simulink model "receiver_overall_reset"  (Simulink 7.5)
settings: Solver=FixedStepDiscrete  SolverMode=SingleTasking  StartTime=0.0  StopTime=(length(simin.signals.values)-1)/Fs  FixedStep=1  RelTol=1e-3
undefined symbols (not defined in the file): Fs
libraries: xbsIndex_r4 x962
(part 1 of 9)
settings Model: Creator=ich  LastModifiedBy=ich
settings DataIOCC: ExternalInput=simin  LimitDataPoints=off  LoadExternalInput=on

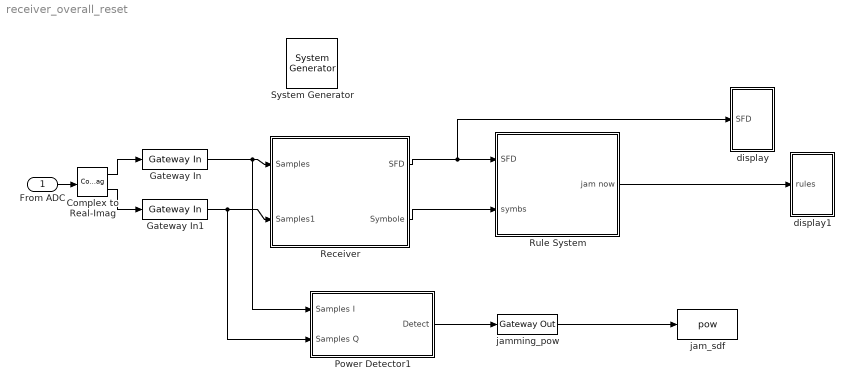
== system receiver_overall_reset ==
  From ADC : Inport  SampleTime=1/Fs  OutDataType=fixdt(1, 16)  OutScaling=2^0  Interpolate=off
      settings: SignalType=complex
  " System Generator" : xbsIndex_r4/ System Generator  Tag=genX  SystemSampleTime=-1  xilinxfamily=spartan3  part=xc3s2000  speed=-5  package=fg456  synthesis_tool=XST  clock_wrapper=Clock Enables  directory=G:/Projekte/wireless_firewall/dschung/IEEE 802.15.4 receiver/receiver_overall_reset  testbench=off  simulink_period=1  sysclk_period=10  dcm_input_clock_period=10  incr_netlist=off  trim_vbits=Everywhere in SubSystem  dbl_ovrd=According to Block Masks  core_generation=According to Block Masks  run_coregen=off  deprecated_control=off  eval_field=0  block_type=sysgen
      settings: block_version=12.1
  Complex to Real-Imag : ComplexToRealImag
  Gateway In : xbsIndex_r4/Gateway In  arith_type="Signed  (2's comp)"  n_bits=15  bin_pt=13  quantization="Round  (unbiased: +/- Inf)"  overflow=Saturate  period=1/Fs  dbl_ovrd=off  timing_constraint=None  locs_specified=off  LOCs={}  hdl_port=on  block_type=gatewayin
      settings: infoedit="Gateway in block.  Converts inputs of type Simulink integer, double and fixed point to  Xilinx fixed point type.<br><br>Hardware notes:  In hardware these blocks become top level input ports."  xl_area=[0 0 0 0 16 0 0]  block_version=12.1
  Gateway In1 : xbsIndex_r4/Gateway In  arith_type="Signed  (2's comp)"  n_bits=15  bin_pt=13  quantization="Round  (unbiased: +/- Inf)"  overflow=Saturate  period=1/Fs  dbl_ovrd=off  timing_constraint=None  locs_specified=off  LOCs={}  hdl_port=on  block_type=gatewayin
      settings: infoedit="Gateway in block.  Converts inputs of type Simulink integer, double and fixed point to  Xilinx fixed point type.<br><br>Hardware notes:  In hardware these blocks become top level input ports."  xl_area=[0 0 0 0 16 0 0]  block_version=12.1
  Power Detector1 : Subsystem
  Receiver : Subsystem
  Rule System : Subsystem  mask{head=4, s16a=0, spl=0, spu=0, s16l=0, s16u=0, d16a=0, dpl=0, dpu=0, d16l=0, d16u=0, b64a=0, d64lr=0, d64ll=0, d64ur=0, d64ul=0, s64lr=0, s64ll=0, s64ur=0, s64ul=0}
      mask prompts: head "Header Jam Type"; s16a "Source 16 bit Address"; spl "Source PAN lower"; spu "Source PAN upper"; s16l "Source 16 bit lower"; s16u "Source 16 bit upper"; d16a "Dest 16bit Address"; dpl "Dest PAN lower"; dpu "Dest PAN upper"; d16l "Dest 16 bit lower"; d16u "Dest 16 bit upper"; b64a "64 bit add jamming"; d64lr "Dest 64 bit lower rigth part"; d64ll "Dest 64 bit lower left part"; d64ur "Dest 64 bit upper rigth part"; d64ul "Dest 64 bit upper left part"; s64lr "Source 64 bit lower rigth part"; s64ll "Source 64 bit lower left part"; s64ur "Source 64 bit upper rigth part"; s64ul "Source 64 bit upper left part"
      mask help:
      | head:
      |   first bit: security
      |   second bit: is Beacon
      |   third bit: is MAC
      | Dest + Source 16 Addresses:
      |   first bit: PAN
      |   second bit: Address
      |  Addresses with MSB rigth!
      | 64 bit Addresses:
      |   first bit: Destination
      |   second bit: Source
      |  Addresses with MSB rigth!
      |  Bsp: 123456789ABCDEFG0 -->
      |    rigth: '87654321'
      |    left:  '0FEDCBA9'
  display : Subsystem
  display1 : Subsystem
  jam_sdf : ToWorkspace  VariableName=pow  SampleTime=-1  SaveFormat=Structure
  jamming_pow : xbsIndex_r4/Gateway Out  hdl_port=on  timing_constraint=None  locs_specified=off  LOCs={}  block_type=gatewayout
      settings: infoedit="Gateway out block.  Converts Xilinx fixed point inputs into ouputs of type Simulink integer, double, or fixed point.<br><br>Hardware notes:  In hardware these blocks become top level output ports or are discarded, depending on how they are configured."  block_version=12.2
  wires:
  Receiver/2(Symbole) -> Rule System/2(symbs)
  Receiver/1(SFD) -> Rule System/1(SFD), display/1(SFD)
  Rule System/1(jam now) -> display1/1(rules)
  Gateway In/1 -> Receiver/1(Samples), Power Detector1/1(Samples I)
  Gateway In1/1 -> Receiver/2(Samples1), Power Detector1/2(Samples Q)
  From ADC/1 -> Complex to Real-Imag/1
  Complex to Real-Imag/1 -> Gateway In/1
  Complex to Real-Imag/2 -> Gateway In1/1
  jamming_pow/1 -> jam_sdf/1
  Power Detector1/1(Detect) -> jamming_pow/1

== system receiver_overall_reset/Power Detector1 ==
  Samples I : Inport
  Samples Q : Inport  Port=2
  -23dB : xbsIndex_r4/Constant  arith_type=Unsigned  const=0.005  n_bits=16  bin_pt=16  explicit_period=off  period=1  equ=P=C  opselect=C  inp2=PCIN>>17  opr=+  inp1=P  carry=CIN  dbl_ovrd=off  block_type=constant
      settings: block_version=12.2
  AddSub : xbsIndex_r4/AddSub  mode=Addition  use_carryin=off  use_carryout=off  en=off  latency=0  precision=Full  arith_type=Unsigned  n_bits=16  bin_pt=14  quantization=Truncate  overflow=Wrap  dbl_ovrd=off  use_behavioral_HDL=off  hw_selection=Fabric  pipelined=off  block_type=addsub
      settings: block_version=12.2
  Moving Average : Subsystem
  Mult : xbsIndex_r4/Mult  precision=User Defined  arith_type=Unsigned  n_bits=28  bin_pt=26  quantization=Truncate  overflow=Wrap  en=off  latency=1  dbl_ovrd=off  use_behavioral_HDL=off  opt=Speed  use_embedded=on  optimum_pipeline=off  pipeline=on  use_rpm=on  placement_style=Triangular  block_type=mult
      settings: block_version=12.2
  Mult1 : xbsIndex_r4/Mult  precision=User Defined  arith_type=Unsigned  n_bits=28  bin_pt=26  quantization=Truncate  overflow=Wrap  en=off  latency=1  dbl_ovrd=off  use_behavioral_HDL=off  opt=Speed  use_embedded=on  optimum_pipeline=off  pipeline=on  use_rpm=on  placement_style=Triangular  block_type=mult
      settings: block_version=12.2
  Relational2 : xbsIndex_r4/Relational  mode=a>b  en=off  latency=1  dbl_ovrd=off  block_type=relational
      settings: block_version=12.2
  Terminator : Terminator
  power-level : xbsIndex_r4/Gateway Out  hdl_port=on  timing_constraint=None  locs_specified=off  LOCs={}  block_type=gatewayout
      settings: infoedit="Gateway out block.  Converts Xilinx fixed point inputs into ouputs of type Simulink integer, double, or fixed point.<br><br>Hardware notes:  In hardware these blocks become top level output ports or are discarded, depending on how they are configured."  block_version=12.2
  Detect : Outport
  wires:
  Samples Q/1 -> Mult1/2, Mult1/1
  Relational2/1 -> Detect/1
  Samples I/1 -> Mult/1, Mult/2
  Mult/1 -> AddSub/1
  Mult1/1 -> AddSub/2
  AddSub/1 -> Moving Average/1(in)
  -23dB/1 -> Relational2/2
  Moving Average/1(short) -> Relational2/1, power-level/1
  power-level/1 -> Terminator/1

== system receiver_overall_reset/Receiver ==
  Samples : Inport
  Samples1 : Inport  Port=2
  CRC : Subsystem
  Delay1 : xbsIndex_r4/Delay  en=off  latency=2  dbl_ovrd=off  reg_retiming=off  block_type=delay
      settings: block_version=12.2
  Delay2 : xbsIndex_r4/Delay  en=off  latency=1  dbl_ovrd=off  reg_retiming=off  block_type=delay
      settings: block_version=12.2
  Delay3 : xbsIndex_r4/Delay  en=off  latency=1  dbl_ovrd=off  reg_retiming=off  block_type=delay
      settings: block_version=12.2
  Down Sample : xbsIndex_r4/Down Sample  sample_ratio=25  sample_phase="Last Value of Frame  (most efficient)"  en=off  latency=1  dbl_ovrd=off  block_type=dsamp
      settings: block_version=12.2
  Down Sample1 : xbsIndex_r4/Down Sample  sample_ratio=25  sample_phase="Last Value of Frame  (most efficient)"  en=off  latency=1  dbl_ovrd=off  block_type=dsamp
      settings: block_version=12.2
  FM demod : Subsystem
      mask Display:
      | disp('FM\ndemod');
      | port_label('input',1,'I');
      | port_label('input',2,'Q');
      | port_label('output',1,'x');
  Inverter1 : xbsIndex_r4/Inverter  en=off  latency=1  dbl_ovrd=off  block_type=inv
      settings: block_version=12.2
  Logical2 : xbsIndex_r4/Logical  logical_function=OR  inputs=2  en=off  latency=0  precision=Full  arith_type=Unsigned  n_bits=16  bin_pt=0  align_bp=on  dbl_ovrd=off  block_type=logical
      settings: block_version=12.2
  Logical4 : xbsIndex_r4/Logical  logical_function=AND  inputs=2  en=off  latency=0  precision=Full  arith_type=Unsigned  n_bits=16  bin_pt=0  align_bp=on  dbl_ovrd=off  block_type=logical
      settings: block_version=12.2
  Logical5 : xbsIndex_r4/Logical  logical_function=AND  inputs=2  en=off  latency=0  precision=Full  arith_type=Unsigned  n_bits=16  bin_pt=0  align_bp=on  dbl_ovrd=off  block_type=logical
      settings: block_version=12.2
  PSDU length : Subsystem
  SFD_d : Subsystem
  Sym-Chooser : Subsystem  mask{thresh=16}
      mask prompts: thresh "Threshold"
  Sym-Clk : Subsystem
  Terminator : Terminator
  Terminator1 : Terminator
  Terminator2 : Terminator
  To Workspace1 : ToWorkspace  VariableName=symbole_clk  SampleTime=-1  SaveFormat=Structure
  To Workspace2 : ToWorkspace  VariableName=symbole  SampleTime=-1  SaveFormat=Structure
  To Workspace3 : ToWorkspace  VariableName=symbole_running  SampleTime=-1  SaveFormat=Structure
  WaveScope : xbsIndex_r4/WaveScope  block_type=wavescope
      settings: block_version=12.2
  sylbole_clk : xbsIndex_r4/Gateway Out  hdl_port=on  timing_constraint=None  locs_specified=off  LOCs={}  block_type=gatewayout
      settings: infoedit="Gateway out block.  Converts Xilinx fixed point inputs into ouputs of type Simulink integer, double, or fixed point.<br><br>Hardware notes:  In hardware these blocks become top level output ports or are discarded, depending on how they are configured."  block_version=12.2
  symbole : xbsIndex_r4/Gateway Out  hdl_port=on  timing_constraint=None  locs_specified=off  LOCs={}  block_type=gatewayout
      settings: infoedit="Gateway out block.  Converts Xilinx fixed point inputs into ouputs of type Simulink integer, double, or fixed point.<br><br>Hardware notes:  In hardware these blocks become top level output ports or are discarded, depending on how they are configured."  block_version=12.2
  symbole_running : xbsIndex_r4/Gateway Out  hdl_port=on  timing_constraint=None  locs_specified=off  LOCs={}  block_type=gatewayout
      settings: infoedit="Gateway out block.  Converts Xilinx fixed point inputs into ouputs of type Simulink integer, double, or fixed point.<br><br>Hardware notes:  In hardware these blocks become top level output ports or are discarded, depending on how they are configured."  block_version=12.2
  to octet : Subsystem
  SFD : Outport  OutDataType=fixdt(1, 16)  OutScaling=2^0
  Symbole : Outport  Port=2
  wires:
  FM demod/1(x) -> Sym-Chooser/1(In), Sym-Clk/1(x)
  Sym-Clk/1(clk) -> Sym-Chooser/2(clk), sylbole_clk/1
  to octet/1(Out) -> SFD_d/2(data), PSDU length/2(data)
  Delay1/1 -> CRC/2(rst), PSDU length/1(now)
  PSDU length/1(length) -> Sym-Clk/2(PSDU length)
  Sym-Clk/2(end) -> CRC/1(now), Logical4/2
  CRC/1(ok) -> Terminator/1
  Sym-Clk/3(not running) -> SFD_d/1(not running)
  Sym-Chooser/2(symb) -> CRC/3(data), Symbole/1, symbole/1, to octet/1(In)
  SFD_d/1(fnd) -> Terminator1/1, SFD/1, Delay1/1, Delay3/1
  Sym-Chooser/1(fnd) -> Terminator2/1
  Samples/1 -> Down Sample/1
  Samples1/1 -> Down Sample1/1
  Down Sample/1 -> FM demod/1(I)
  Down Sample1/1 -> FM demod/2(Q)
  symbole/1 -> To Workspace2/1
  sylbole_clk/1 -> To Workspace1/1
  symbole_running/1 -> To Workspace3/1
  Delay2/1 -> Logical2/2
  Logical2/1 -> Logical5/1
  Inverter1/1 -> Logical5/2
  Logical5/1 -> Delay2/1, Logical4/1, symbole_running/1
  Logical4/1 -> Inverter1/1
  Delay3/1 -> Logical2/1

== system receiver_overall_reset/Rule System ==
  SFD : Inport
  symbs : Inport  Port=2
  16bit Addresses + PANs : Subsystem
  64 bit Settings : xbsIndex_r4/Constant  arith_type=Unsigned  const=b64a  n_bits=2  bin_pt=0  explicit_period=off  period=1  equ=P=C  opselect=C  inp2=PCIN>>17  opr=+  inp1=P  carry=CIN  dbl_ovrd=off  block_type=constant
      settings: block_version=12.2
  64bit Addresses : Subsystem
  Concat : xbsIndex_r4/Concat  num_inputs=4  dbl_ovrd=off  block_type=concat
      settings: block_version=12.2
  Constant : xbsIndex_r4/Constant  arith_type=Unsigned  const=0  n_bits=16  bin_pt=0  explicit_period=off  period=1  equ=P=C  opselect=C  inp2=PCIN>>17  opr=+  inp1=P  carry=CIN  dbl_ovrd=off  block_type=constant
      settings: block_version=12.2
  Delay1 : xbsIndex_r4/Delay  en=off  latency=1  dbl_ovrd=off  reg_retiming=off  block_type=delay
      settings: block_version=12.2
  Delay2 : xbsIndex_r4/Delay  en=off  latency=6  dbl_ovrd=off  reg_retiming=off  block_type=delay
      settings: block_version=12.2
  Delay6 : xbsIndex_r4/Delay  en=off  latency=1  dbl_ovrd=off  reg_retiming=off  block_type=delay
      settings: block_version=12.2
  Delay7 : xbsIndex_r4/Delay  en=off  latency=1  dbl_ovrd=off  reg_retiming=off  block_type=delay
      settings: block_version=12.2
  Dest 16 Settings : xbsIndex_r4/Constant  arith_type=Unsigned  const=d16a  n_bits=2  bin_pt=0  explicit_period=off  period=1  equ=P=C  opselect=C  inp2=PCIN>>17  opr=+  inp1=P  carry=CIN  dbl_ovrd=off  block_type=constant
      settings: block_version=12.2
  Gateway Header Out : xbsIndex_r4/Gateway Out  hdl_port=on  timing_constraint=None  locs_specified=off  LOCs={}  block_type=gatewayout
      settings: infoedit="Gateway out block.  Converts Xilinx fixed point inputs into ouputs of type Simulink integer, double, or fixed point.<br><br>Hardware notes:  In hardware these blocks become top level output ports or are discarded, depending on how they are configured."  xl_area=[0 0 0 0 4 0 0]  block_version=12.1
  Gateway longAdd1 : xbsIndex_r4/Gateway Out  hdl_port=on  timing_constraint=None  locs_specified=off  LOCs={}  block_type=gatewayout
      settings: infoedit="Gateway out block.  Converts Xilinx fixed point inputs into ouputs of type Simulink integer, double, or fixed point.<br><br>Hardware notes:  In hardware these blocks become top level output ports or are discarded, depending on how they are configured."  xl_area=[0 0 0 0 4 0 0]  block_version=12.1
  Gateway longAdd2 : xbsIndex_r4/Gateway Out  hdl_port=on  timing_constraint=None  locs_specified=off  LOCs={}  block_type=gatewayout
      settings: infoedit="Gateway out block.  Converts Xilinx fixed point inputs into ouputs of type Simulink integer, double, or fixed point.<br><br>Hardware notes:  In hardware these blocks become top level output ports or are discarded, depending on how they are configured."  xl_area=[0 0 0 0 4 0 0]  block_version=12.1
  Header Analyser : Subsystem
  Logical : xbsIndex_r4/Logical  logical_function=OR  inputs=8  en=off  latency=0  precision=Full  arith_type=Unsigned  n_bits=16  bin_pt=0  align_bp=on  dbl_ovrd=off  block_type=logical
      settings: block_version=12.2
  Mux1 : xbsIndex_r4/Mux  inputs=2  en=off  latency=0  precision=Full  arith_type=Unsigned  n_bits=16  bin_pt=14  quantization=Truncate  overflow=Wrap  dbl_ovrd=off  block_type=mux
      settings: block_version=12.2
  Source 16b Settings : xbsIndex_r4/Constant  arith_type=Unsigned  const=s16a  n_bits=2  bin_pt=0  explicit_period=off  period=1  equ=P=C  opselect=C  inp2=PCIN>>17  opr=+  inp1=P  carry=CIN  dbl_ovrd=off  block_type=constant
      settings: block_version=12.2
  To Workspace1 : ToWorkspace  VariableName=simout_header  SampleTime=-1  SaveFormat=Array
  To Workspace3 : ToWorkspace  VariableName=longadd_pt1  SampleTime=-1  SaveFormat=Array
  To Workspace4 : ToWorkspace  VariableName=longadd_pt2  SampleTime=-1  SaveFormat=Array
  header : xbsIndex_r4/Constant  arith_type=Unsigned  const=head  n_bits=3  bin_pt=0  explicit_period=off  period=1  equ=P=C  opselect=C  inp2=PCIN>>17  opr=+  inp1=P  carry=CIN  dbl_ovrd=off  block_type=constant
      settings: block_version=12.2
  jam now : Outport  OutDataType=fixdt(1, 16)  OutScaling=2^0
  wires:
  SFD/1 -> Delay2/1
  Delay2/1 -> Header Analyser/2(SFD ind), Mux1/1
  symbs/1 -> Delay1/1, Concat/1
  Concat/1 -> 16bit Addresses + PANs/1(Concat Symbols), 64bit Addresses/1(Concat Symbols), Header Analyser/1(Frame Control), Mux1/3
  Gateway Header Out/1 -> To Workspace1/1
  Gateway longAdd1/1 -> To Workspace3/1
  Gateway longAdd2/1 -> To Workspace4/1
  Header Analyser/2(Dest Add Mode) -> 16bit Addresses + PANs/2(Dest Add Type), 64bit Addresses/2(Dest Add Type)
  Header Analyser/3(Source Add Mode) -> 64bit Addresses/3(Source Add Type), 16bit Addresses + PANs/3(Source Add Type)
  64bit Addresses/1(Add Low) -> Gateway longAdd1/1
  64bit Addresses/2(Add High) -> Gateway longAdd2/1
  Mux1/1 -> Gateway Header Out/1
  Constant/1 -> Mux1/2
  Header Analyser/1(jam type) -> Logical/1
  16bit Addresses + PANs/1(jam Dest Address) -> Logical/2
  16bit Addresses + PANs/2(jam Source Address) -> Logical/3
  16bit Addresses + PANs/3(jam Dest Pan) -> Logical/4
  64bit Addresses/3(Dest 64b Jam) -> Logical/6
  64bit Addresses/4(Source 64b Jam) -> Logical/7
  Logical/1 -> jam now/1
  Delay6/1 -> Concat/3, Delay7/1
  Delay7/1 -> Concat/4
  Delay1/1 -> Concat/2, Delay6/1
  Header Analyser/4(jam Security) -> Logical/8
  header/1 -> Header Analyser/3(Header Settings)
  Dest 16 Settings/1 -> 16bit Addresses + PANs/5(Destination Settings)
  Source 16b Settings/1 -> 16bit Addresses + PANs/4(Source Settings)
  64 bit Settings/1 -> 64bit Addresses/4(Address 64b Settings)
  16bit Addresses + PANs/4(jam Source Pan) -> Logical/5

== system receiver_overall_reset/display ==
  SFD : Inport
  Constant : xbsIndex_r4/Constant  arith_type=Unsigned  const=2^17  n_bits=18  bin_pt=0  explicit_period=off  period=1  equ=P=C  opselect=C  inp2=PCIN>>17  opr=+  inp1=P  carry=CIN  dbl_ovrd=off  block_type=constant
      settings: block_version=12.2
  Counter : xbsIndex_r4/Counter  cnt_type=Free Running  cnt_to=Inf  operation=Up  start_count=0  cnt_by_val=1  arith_type=Unsigned  n_bits=18  bin_pt=0  load_pin=off  rst=off  en=off  explicit_period=on  period=1600  dbl_ovrd=off  use_behavioral_HDL=off  implementation=Fabric  block_type=counter
      settings: block_version=12.2
  Counter_paket : xbsIndex_r4/Counter  cnt_type=Free Running  cnt_to=Inf  operation=Up  start_count=0  cnt_by_val=1  arith_type=Unsigned  n_bits=10  bin_pt=0  load_pin=off  rst=off  en=on  explicit_period=off  period=1  dbl_ovrd=off  use_behavioral_HDL=off  implementation=Fabric  block_type=counter
      settings: block_version=12.2
  Mux : xbsIndex_r4/Mux  inputs=2  en=off  latency=0  precision=Full  arith_type=Unsigned  n_bits=16  bin_pt=14  quantization=Truncate  overflow=Wrap  dbl_ovrd=off  block_type=mux
      settings: block_version=12.2
  Relational : xbsIndex_r4/Relational  mode=a>b  en=off  latency=0  dbl_ovrd=off  block_type=relational
      settings: block_version=12.2
  Slice : xbsIndex_r4/Slice  nbits=5  boolean_output=off  mode=Lower Bit Location + Width  bit1=0  base1=MSB of Input  bit0=0  base0=LSB of Input  dbl_ovrd=off  block_type=slice
      settings: block_version=12.2
  Slice1 : xbsIndex_r4/Slice  nbits=5  boolean_output=off  mode=Upper Bit Location + Width  bit1=0  base1=MSB of Input  bit0=0  base0=LSB of Input  dbl_ovrd=off  block_type=slice
      settings: block_version=12.2
  Up Sample : xbsIndex_r4/Up Sample  sample_ratio=1600  copy_samples=off  en=off  latency=0  dbl_ovrd=off  block_type=usamp
      settings: block_version=12.2
  count_sdf : ToWorkspace  VariableName=count_sdf  SampleTime=-1  SaveFormat=Structure
  count_sdf1 : ToWorkspace  VariableName=count_sdf1  SampleTime=-1  SaveFormat=Structure
  counter_sfd : xbsIndex_r4/Gateway Out  hdl_port=on  timing_constraint=None  locs_specified=off  LOCs={}  block_type=gatewayout
      settings: infoedit="Gateway out block.  Converts Xilinx fixed point inputs into ouputs of type Simulink integer, double, or fixed point.<br><br>Hardware notes:  In hardware these blocks become top level output ports or are discarded, depending on how they are configured."  block_version=12.2
  jam_sdf : ToWorkspace  VariableName=js  SampleTime=-1  SaveFormat=Structure
  jamming_sfd : xbsIndex_r4/Gateway Out  hdl_port=on  timing_constraint=None  locs_specified=off  LOCs={}  block_type=gatewayout
      settings: infoedit="Gateway out block.  Converts Xilinx fixed point inputs into ouputs of type Simulink integer, double, or fixed point.<br><br>Hardware notes:  In hardware these blocks become top level output ports or are discarded, depending on how they are configured."  block_version=12.2
  select : xbsIndex_r4/Gateway Out  hdl_port=on  timing_constraint=None  locs_specified=off  LOCs={}  block_type=gatewayout
      settings: infoedit="Gateway out block.  Converts Xilinx fixed point inputs into ouputs of type Simulink integer, double, or fixed point.<br><br>Hardware notes:  In hardware these blocks become top level output ports or are discarded, depending on how they are configured."  block_version=12.2
  wires:
  counter_sfd/1 -> count_sdf/1
  SFD/1 -> Counter_paket/1, Up Sample/1
  jamming_sfd/1 -> jam_sdf/1
  Counter_paket/1 -> Slice/1, Slice1/1
  Mux/1 -> counter_sfd/1
  Slice1/1 -> Mux/3
  Slice/1 -> Mux/2
  Counter/1 -> Relational/1
  Constant/1 -> Relational/2
  select/1 -> count_sdf1/1
  Relational/1 -> select/1, Mux/1
  Up Sample/1 -> jamming_sfd/1

== system receiver_overall_reset/display1 ==
  rules : Inport
  Constant : xbsIndex_r4/Constant  arith_type=Unsigned  const=2^17  n_bits=18  bin_pt=0  explicit_period=off  period=1  equ=P=C  opselect=C  inp2=PCIN>>17  opr=+  inp1=P  carry=CIN  dbl_ovrd=off  block_type=constant
      settings: block_version=12.2
  Counter : xbsIndex_r4/Counter  cnt_type=Free Running  cnt_to=Inf  operation=Up  start_count=0  cnt_by_val=1  arith_type=Unsigned  n_bits=18  bin_pt=0  load_pin=off  rst=off  en=off  explicit_period=on  period=1600  dbl_ovrd=off  use_behavioral_HDL=off  implementation=Fabric  block_type=counter
      settings: block_version=12.2
  Counter_paket : xbsIndex_r4/Counter  cnt_type=Free Running  cnt_to=Inf  operation=Up  start_count=0  cnt_by_val=1  arith_type=Unsigned  n_bits=10  bin_pt=0  load_pin=off  rst=off  en=on  explicit_period=off  period=1  dbl_ovrd=off  use_behavioral_HDL=off  implementation=Fabric  block_type=counter
      settings: block_version=12.2
  Mux : xbsIndex_r4/Mux  inputs=2  en=off  latency=0  precision=Full  arith_type=Unsigned  n_bits=16  bin_pt=14  quantization=Truncate  overflow=Wrap  dbl_ovrd=off  block_type=mux
      settings: block_version=12.2
  Relational : xbsIndex_r4/Relational  mode=a>b  en=off  latency=0  dbl_ovrd=off  block_type=relational
      settings: block_version=12.2
  Slice : xbsIndex_r4/Slice  nbits=5  boolean_output=off  mode=Lower Bit Location + Width  bit1=0  base1=MSB of Input  bit0=0  base0=LSB of Input  dbl_ovrd=off  block_type=slice
      settings: block_version=12.2
  Slice1 : xbsIndex_r4/Slice  nbits=5  boolean_output=off  mode=Upper Bit Location + Width  bit1=0  base1=MSB of Input  bit0=0  base0=LSB of Input  dbl_ovrd=off  block_type=slice
      settings: block_version=12.2
  Up Sample : xbsIndex_r4/Up Sample  sample_ratio=1600  copy_samples=off  en=off  latency=0  dbl_ovrd=off  block_type=usamp
      settings: block_version=12.2
  count_sdf : ToWorkspace  VariableName=count_r  SampleTime=-1  SaveFormat=Structure
  count_sdf1 : ToWorkspace  VariableName=select_r  SampleTime=-1  SaveFormat=Structure
  counter_r : xbsIndex_r4/Gateway Out  hdl_port=on  timing_constraint=None  locs_specified=off  LOCs={}  block_type=gatewayout
      settings: infoedit="Gateway out block.  Converts Xilinx fixed point inputs into ouputs of type Simulink integer, double, or fixed point.<br><br>Hardware notes:  In hardware these blocks become top level output ports or are discarded, depending on how they are configured."  block_version=12.2
  jam_sdf : ToWorkspace  VariableName=jr  SampleTime=-1  SaveFormat=Structure
  jamming_r : xbsIndex_r4/Gateway Out  hdl_port=on  timing_constraint=None  locs_specified=off  LOCs={}  block_type=gatewayout
      settings: infoedit="Gateway out block.  Converts Xilinx fixed point inputs into ouputs of type Simulink integer, double, or fixed point.<br><br>Hardware notes:  In hardware these blocks become top level output ports or are discarded, depending on how they are configured."  block_version=12.2
  select_r : xbsIndex_r4/Gateway Out  hdl_port=on  timing_constraint=None  locs_specified=off  LOCs={}  block_type=gatewayout
      settings: infoedit="Gateway out block.  Converts Xilinx fixed point inputs into ouputs of type Simulink integer, double, or fixed point.<br><br>Hardware notes:  In hardware these blocks become top level output ports or are discarded, depending on how they are configured."  block_version=12.2
  wires:
  counter_r/1 -> count_sdf/1
  rules/1 -> Counter_paket/1, Up Sample/1
  jamming_r/1 -> jam_sdf/1
  Counter_paket/1 -> Slice/1, Slice1/1
  Mux/1 -> counter_r/1
  Slice1/1 -> Mux/3
  Slice/1 -> Mux/2
  Counter/1 -> Relational/1
  Constant/1 -> Relational/2
  select_r/1 -> count_sdf1/1
  Relational/1 -> select_r/1, Mux/1
  Up Sample/1 -> jamming_r/1

== system receiver_overall_reset/Power Detector1/Moving Average ==
  in : Inport
  AddSub1 : xbsIndex_r4/AddSub  mode=Addition  use_carryin=off  use_carryout=off  en=off  latency=1  precision=User Defined  arith_type=Unsigned  n_bits=39  bin_pt=31  quantization=Truncate  overflow=Wrap  dbl_ovrd=off  use_behavioral_HDL=off  hw_selection=Fabric  pipelined=off  block_type=addsub
      settings: block_version=12.2
  AddSub2 : xbsIndex_r4/AddSub  mode=Subtraction  use_carryin=off  use_carryout=off  en=off  latency=0  precision=Full  arith_type=Unsigned  n_bits=16  bin_pt=14  quantization=Truncate  overflow=Wrap  dbl_ovrd=off  use_behavioral_HDL=off  hw_selection=Fabric  pipelined=off  block_type=addsub
      settings: block_version=12.2
  Convert : xbsIndex_r4/Convert  arith_type="Signed  (2's comp)"  n_bits=31  bin_pt=26  quantization=Truncate  overflow=Wrap  en=off  latency=0  dbl_ovrd=off  pipeline=off  block_type=convert
      settings: block_version=12.2
  Convert1 : xbsIndex_r4/Convert  arith_type=Unsigned  n_bits=32  bin_pt=30  quantization=Truncate  overflow=Wrap  en=off  latency=0  dbl_ovrd=off  pipeline=off  block_type=convert
      settings: block_version=12.2
  Delay1 : xbsIndex_r4/Delay  en=off  latency=32  dbl_ovrd=off  reg_retiming=off  block_type=delay
      settings: block_version=12.2
  Down Sample : xbsIndex_r4/Down Sample  sample_ratio=6  sample_phase="Last Value of Frame  (most efficient)"  en=off  latency=1  dbl_ovrd=off  block_type=dsamp
      settings: block_version=12.2
  Reinterpret : xbsIndex_r4/Reinterpret  force_arith_type=off  arith_type=Unsigned  force_bin_pt=on  bin_pt=31  block_type=reinterpret
      settings: infoedit="Changes signal type without altering the binary representation.   You can changed the signal between signed and unsigned, and relocate the binary point.<br><br>Hardware notes: In hardware this block costs nothing.<br><br>Example:  Suppose the input is 6 bits wide, signed, with 2 fractional bits, and the output is forced to unsigned with 0 fractional bits.  Then an input of -2.0 (1110.00 in binary 2's complement) becomes an output of 56 (111000 in binary)."  block_version=12.2
  Up Sample : xbsIndex_r4/Up Sample  sample_ratio=6  copy_samples=on  en=off  latency=0  dbl_ovrd=off  block_type=usamp
      settings: block_version=12.2
  short : Outport
  wires:
  in/1 -> Down Sample/1
  Delay1/1 -> AddSub2/2
  AddSub2/1 -> Convert/1
  AddSub1/1 -> Up Sample/1, AddSub1/2
  Reinterpret/1 -> AddSub1/1
  Down Sample/1 -> Delay1/1, AddSub2/1
  Up Sample/1 -> Convert1/1
  Convert/1 -> Reinterpret/1
  Convert1/1 -> short/1

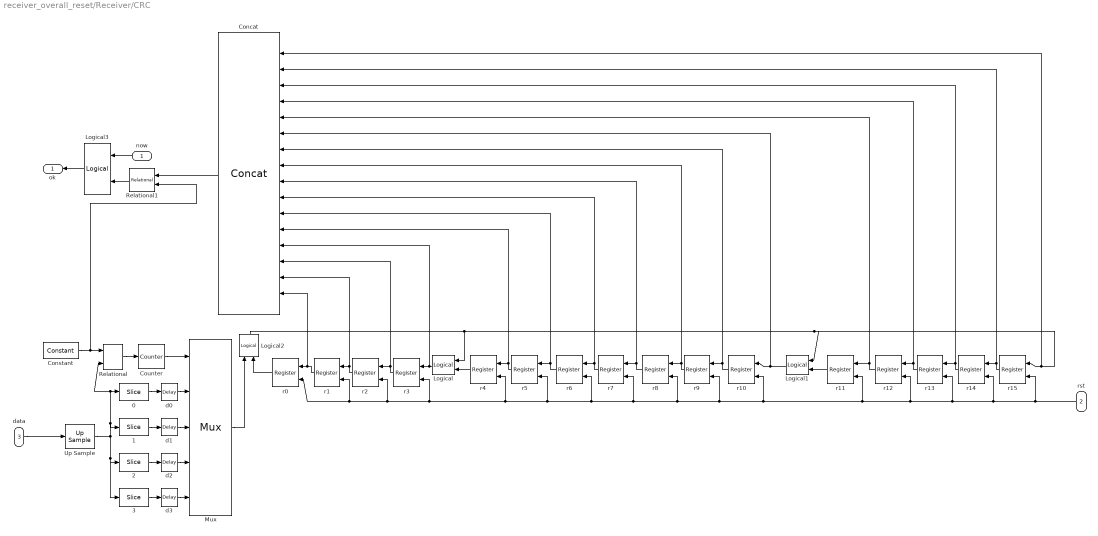
== system receiver_overall_reset/Receiver/CRC ==
  now : Inport  OutDataType=fixdt(1, 16)  OutScaling=2^0
  rst : Inport  Port=2
  data : Inport  Port=3
  0 : xbsIndex_r4/Slice  nbits=1  boolean_output=off  mode=Lower Bit Location + Width  bit1=0  base1=MSB of Input  bit0=0  base0=LSB of Input  dbl_ovrd=off  block_type=slice
      settings: block_version=12.2
  1 : xbsIndex_r4/Slice  nbits=1  boolean_output=off  mode=Lower Bit Location + Width  bit1=0  base1=MSB of Input  bit0=1  base0=LSB of Input  dbl_ovrd=off  block_type=slice
      settings: block_version=12.2
  2 : xbsIndex_r4/Slice  nbits=1  boolean_output=off  mode=Lower Bit Location + Width  bit1=0  base1=MSB of Input  bit0=2  base0=LSB of Input  dbl_ovrd=off  block_type=slice
      settings: block_version=12.2
  3 : xbsIndex_r4/Slice  nbits=1  boolean_output=off  mode=Lower Bit Location + Width  bit1=0  base1=MSB of Input  bit0=3  base0=LSB of Input  dbl_ovrd=off  block_type=slice
      settings: block_version=12.2
  Concat : xbsIndex_r4/Concat  num_inputs=16  dbl_ovrd=off  block_type=concat
      settings: block_version=12.2
  Constant : xbsIndex_r4/Constant  arith_type=Unsigned  const=0  n_bits=1  bin_pt=0  explicit_period=off  period=1  equ=P=C  opselect=C  inp2=PCIN>>17  opr=+  inp1=P  carry=CIN  dbl_ovrd=off  block_type=constant
      settings: block_version=12.2
  Counter : xbsIndex_r4/Counter  cnt_type=Free Running  cnt_to=Inf  operation=Up  start_count=0  cnt_by_val=1  arith_type=Unsigned  n_bits=2  bin_pt=0  load_pin=off  rst=on  en=off  explicit_period=off  period=1  dbl_ovrd=off  use_behavioral_HDL=off  implementation=Fabric  block_type=counter
      settings: block_version=12.2
  Logical : xbsIndex_r4/Logical  logical_function=XOR  inputs=2  en=off  latency=0  precision=Full  arith_type=Unsigned  n_bits=16  bin_pt=0  align_bp=on  dbl_ovrd=off  block_type=logical
      settings: block_version=12.2
  Logical1 : xbsIndex_r4/Logical  logical_function=XOR  inputs=2  en=off  latency=0  precision=Full  arith_type=Unsigned  n_bits=16  bin_pt=0  align_bp=on  dbl_ovrd=off  block_type=logical
      settings: block_version=12.2
  Logical2 : xbsIndex_r4/Logical  logical_function=XOR  inputs=2  en=off  latency=0  precision=Full  arith_type=Unsigned  n_bits=16  bin_pt=0  align_bp=on  dbl_ovrd=off  block_type=logical
      settings: block_version=12.2
  Logical3 : xbsIndex_r4/Logical  logical_function=AND  inputs=2  en=off  latency=0  precision=Full  arith_type=Unsigned  n_bits=16  bin_pt=0  align_bp=on  dbl_ovrd=off  block_type=logical
      settings: block_version=12.2
  Mux : xbsIndex_r4/Mux  inputs=4  en=off  latency=0  precision=Full  arith_type=Unsigned  n_bits=16  bin_pt=14  quantization=Truncate  overflow=Wrap  dbl_ovrd=off  block_type=mux
      settings: block_version=12.2
  Relational : xbsIndex_r4/Relational  mode=a!=b  en=off  latency=0  dbl_ovrd=off  block_type=relational
      settings: block_version=12.2
  Relational1 : xbsIndex_r4/Relational  mode=a=b  en=off  latency=0  dbl_ovrd=off  block_type=relational
      settings: block_version=12.2
  Up Sample : xbsIndex_r4/Up Sample  sample_ratio=4  copy_samples=off  en=off  latency=0  dbl_ovrd=off  block_type=usamp
      settings: block_version=12.2
  d0 : xbsIndex_r4/Delay  en=off  latency=1  dbl_ovrd=off  reg_retiming=off  block_type=delay
      settings: block_version=12.2
  d1 : xbsIndex_r4/Delay  en=off  latency=2  dbl_ovrd=off  reg_retiming=off  block_type=delay
      settings: block_version=12.2
  d2 : xbsIndex_r4/Delay  en=off  latency=3  dbl_ovrd=off  reg_retiming=off  block_type=delay
      settings: block_version=12.2
  d3 : xbsIndex_r4/Delay  en=off  latency=4  dbl_ovrd=off  reg_retiming=off  block_type=delay
      settings: block_version=12.2
  r{0..15} (16 alike) : xbsIndex_r4/Register  init=0  rst=on  en=off  dbl_ovrd=off  block_type=register
      settings: block_version=12.2
  ok : Outport  OutDataType=fixdt(1, 16)  OutScaling=2^0
  wires:
  Logical1/1 -> r10/1, Concat/6
  r4/1 -> Logical/2
  Logical2/1 -> Logical1/1, r15/1, Concat/1, Logical/1
  Up Sample/1 -> 1/1, 0/1, Relational/2, 2/1, 3/1
  data/1 -> Up Sample/1
  3/1 -> d3/1
  0/1 -> d0/1
  1/1 -> d1/1
  2/1 -> d2/1
  Mux/1 -> Logical2/1
  Counter/1 -> Mux/1
  Relational/1 -> Counter/1
  Constant/1 -> Relational/1, Relational1/2
  d1/1 -> Mux/3
  d2/1 -> Mux/4
  d3/1 -> Mux/5
  d0/1 -> Mux/2
  Logical/1 -> r3/1, Concat/13
  r3/1 -> r2/1, Concat/14
  r2/1 -> r1/1, Concat/15
  r1/1 -> r0/1, Concat/16
  r0/1 -> Logical2/2
  r10/1 -> r9/1, Concat/7
  r9/1 -> r8/1, Concat/8
  r8/1 -> r7/1, Concat/9
  r7/1 -> r6/1, Concat/10
  r6/1 -> r5/1, Concat/11
  r5/1 -> r4/1, Concat/12
  r11/1 -> Logical1/2
  r12/1 -> r11/1, Concat/5
  r13/1 -> r12/1, Concat/4
  r14/1 -> r13/1, Concat/3
  r15/1 -> r14/1, Concat/2
  rst/1 -> r0/2, r1/2, r2/2, r3/2, r4/2, r5/2, r6/2, r7/2, r8/2, r9/2, r10/2, r11/2, r12/2, r13/2, r14/2, r15/2
  Concat/1 -> Relational1/1
  Relational1/1 -> Logical3/2
  now/1 -> Logical3/1
  Logical3/1 -> ok/1

== system receiver_overall_reset/Receiver/FM demod ==
  I : Inport
  Q : Inport  Port=2
  CORDIC ATAN : Subsystem  mask(Xilinx CORDIC ATAN){stages=5, pe_nbits=33, pe_binpt=28, pipeline_x=ones(1,8), prev_stages=5, pipeline=[1  1  1  1  1]}
      mask prompts: stages "Number of Processing Elements (integer value starting from 1)"; pe_nbits "X, Y Data Width"; pe_binpt "X, Y Binary Point Position"; pipeline_x "Latency for each Processing Element [1 0 0 1]"; prev_stages "Previous Number of Stages"; pipeline "Previous Pipeline Values"
      mask help: A parallel implementation, circular vectoring mode CORDIC processor for performing rectangular-to-polar conversion. The number of iteration stages (and resultant output accuracy) and the processor arithmetic precision are controlled by the mask customization.
      mask init:
      | [bg,fg] = xlcmap('XBlock',0);
      | iPos = get_param(gcb,'Position');
      | iWidth=iPos(3)-iPos(1); iHeight=iPos(4)-iPos(2);
      | iCx=iWidth/2;
      | iCy=iHeight/2;
      | [logoX, logoY] = xlogo(iPos);
      | sav_gcb=gcb;
      | stages = round(sum(abs(stages)));
      | if (stages == 0)
      | 	stages = prev_stages;
      | end
      | x = zeros(1,stages);
      | pipe_size = max(size(pipeline_x));
      | if pipe_size >= stages
      | 	x(1,1:stages) = pipeline_x(1,1:stages);
      | else
      | 	x(1,1:pipe_size) = pipeline_x(1,1:pipe_size);
      | end
      | 
      | if (stages ~=prev_stages)
      | 	pipeline=x;
      | 	cordic_pe = find_system(gcb, 'lookUnderMasks', 'all', 'FollowLinks','on','masktype', 'CORDIC parallel PE');
      |     
      |   a=find_system(cordic_pe{1}, 'lookUnderMasks', 'all', 'FollowLinks','on','masktype', 'CORDIC iteration PE');
      |   for i= 2:length(a)
      |     for j=1:3
      | 	  delete_line(cordic_pe{1}, ['CORDIC PE' int2str(i-1) '/' int2str(j)], ['CORDIC PE' int2str(i) '/' int2str(j)]);
      |     end
      |   end
      |     if length(a)>0,
      |       delete_line(cordic_pe{1}, 'x/1', 'CORDIC PE1/1');
      |       delete_line(cordic_pe{1}, 'y/1', 'CORDIC PE1/2');
      |       delete_line(cordic_pe{1}, 'z/1', 'CORDIC PE1/3');
      |       delete_line(cordic_pe{1}, ['CORDIC PE' int2str(length(a)) '/1'],'X/1');
      |       delete_line(cordic_pe{1}, ['CORDIC PE' int2str(length(a)) '/2'],'Terminator/1');
      |       delete_line(cordic_pe{1}, ['CORDIC PE' int2str(length(a)) '/3'],'Z/1');
      |     elseif length(a)==0
      |       temp_port=get_param([cordic_pe{1} '/x'],'porthandles');
      |       temp_line=get_param(temp_port.Outport,'line');
      |       if temp_line>=0  delete_line(temp_line); end
      |       temp_port=get_param([cordic_pe{1} '/y'],'porthandles');
      |       temp_line=get_param(temp_port.Outport,'line');
      |       if temp_line>=0  delete_line(temp_line); end
      |       temp_port=get_param([cordic_pe{1} '/z'],'porthandles');
      |       temp_line=get_param(temp_port.Outport,'line');
      |       if temp_line>=0  delete_line(temp_line); end
      |     end
      | 
      |     for i=2:length(a)
      |       delete_block(a{i});
      |     end
      |     for i=2:stages,
      |         add_block([cordic_pe{1} '/CORDIC PE1'], [cordic_pe{1} '/CORDIC PE' int2str(i)], 'ii', int2str(i-1),'pe_nbits', 'pe_nbits','pe_binpt', 'pe_binpt','pipeline',['pipeline(1,' int2str(i) ')'],'position',[150+(i-1)*125, 70, 205+(i-1)*125, 130]);
      |     end
      | 
      |     for i= 2:stages,
      |       for j=1:3
      | 		add_line(cordic_pe{1}, ['CORDIC PE' int2str(i-1) '/' int2str(j)], ['CORDIC PE' int2str(i) '/' int2str(j)], 'autorouting', 'on');
      |       end
      |     end
      | 
      |     if stages==0
      |       add_line(cordic_pe{1}, 'x/1', 'X/1', 'autorouting', 'on');
      |       add_line(cordic_pe{1}, 'y/1', 'Terminator/1', 'autorouting', 'on');
      |       add_line(cordic_pe{1}, 'z/1', 'Z/1', 'autorouting', 'on');
      |     elseif stages>0
      |       add_line(cordic_pe{1}, 'x/1', 'CORDIC PE1/1', 'autorouting', 'on');
      |       add_line(cordic_pe{1}, 'y/1', 'CORDIC PE1/2', 'autorouting', 'on');
      |       add_line(cordic_pe{1}, 'z/1', 'CORDIC PE1/3', 'autorouting', 'on');
      | 
      |       set_param([cordic_pe{1} '/' 'X'], 'Position', [150+stages*125, 72, 180+stages*125, 86]);
      |       set_param([cordic_pe{1} '/' 'Terminator'], 'Position', [210+stages*125, 92, 225+stages*125, 108]);
      |       set_param([cordic_pe{1} '/' 'Z'], 'Position', [240+stages*125, 113, 270+stages*125, 127]);
      | 
      |       add_line(cordic_pe{1}, ['CORDIC PE' int2str(stages) '/1'], 'X/1', 'autorouting', 'on');
      |       add_line(cordic_pe{1}, ['CORDIC PE' int2str(stages) '/2'], 'Terminator/1', 'autorouting', 'on');
      |       add_line(cordic_pe{1}, ['CORDIC PE' int2str(stages) '/3'],'Z/1', 'autorouting', 'on');
      | 
      |       % force a "compile" of the constituent constant blocks to
      |       % workaround a data propagation problem
      |       find_system(cordic_pe{1}, 'lookUnderMasks', 'all', 'FollowLinks', 'on', 'MaskType','Xilinx Constant Block');
      |   end
      | 	set_param(sav_gcb, 'prev_stages', int2str(stages));
      | 	set_param(sav_gcb, 'pipeline', [ '[' int2str(x) ']']);
      | else
      | 	if (sum(pipeline~=x))
      | 		set_param(gcb, 'pipeline', [ '[' int2str(x) ']']);
      | 	end
      | end
      | str = sprintf('-%d',sum(x) + 3);
      settings: CopyFcn=set_param(gcb, 'MaskSelfModifiable', 'on', 'LinkStatus', 'none');
      mask Help: eval('');xlDoc('-book','sysgen','-topic','CORDIC_ATAN');
      mask Display:
      | patch([0 iWidth iWidth 0],[0 0 iHeight iHeight] , bg);
      | patch(logoX,logoY , fg);
      | text(iCx-6,iCy,'z');
      | text(iCx,iCy+4,str);
      | port_label('input',1,'I');
      | port_label('input',2,'Q');
      | port_label('output',1,'mag');
      | port_label('output',2,'atan');
      | plot([0 0 iWidth iWidth 0], [0 iHeight iHeight 0 0]);
  "Complex Multiplier 3.1 " : xbsIndex_r4/Complex Multiplier 3.1   multtype=Use_Mults  optimizegoal=Performance  outputwidthhigh=32  outputwidthlow=0  latency=-1  roundmode=Truncate  clockenable=off  syncclear=off  ip_name=Complex Multiplier  ip_version=3.1  dsptool_ready=true  ipcore_usecache=true  ipcore_useipmodelcache=true  ipcore_verbose=false  ipcore_latency_parameter='latency'  wrapper_available=true  port_translation_map={ 'ce' => 'en', 'sclr' => 'rst' }  structural_sim=false  block_type=cmpy_v3_1
      settings: xl_use_area=on  xl_area=[600 1053 0 1053 0 0 0]  block_version=12.1
  Delay : xbsIndex_r4/Delay  en=off  latency=1  dbl_ovrd=off  reg_retiming=off  block_type=delay
      settings: xl_area=[8 16 0 0 0 0 0]  block_version=12.1
  Delay1 : xbsIndex_r4/Delay  en=off  latency=1  dbl_ovrd=off  reg_retiming=off  block_type=delay
      settings: xl_area=[8 16 0 0 0 0 0]  block_version=12.1
  Down Sample : xbsIndex_r4/Down Sample  sample_ratio=2  sample_phase="Last Value of Frame  (most efficient)"  en=off  latency=1  dbl_ovrd=off  block_type=dsamp
      settings: xl_area=[1 1 0 0 0 0 0]  block_version=12.1
  Inverter : xbsIndex_r4/Inverter  en=off  latency=0  dbl_ovrd=off  block_type=inv
      settings: xl_area=[0 0 0 0 0 0 0]  block_version=12.1
  MSB : xbsIndex_r4/Slice  nbits=1  boolean_output=off  mode=Upper Bit Location + Width  bit1=0  base1=MSB of Input  bit0=0  base0=LSB of Input  dbl_ovrd=off  block_type=slice
      settings: block_version=12.1
  Negate : xbsIndex_r4/Negate  precision=User Defined  arith_type="Signed  (2's comp)"  n_bits=15  bin_pt=13  quantization=Truncate  overflow=Wrap  en=off  latency=0  dbl_ovrd=off  block_type=negate
      settings: xl_area=[8 0 0 16 0 0 0]  block_version=12.1
  Terminator : Terminator
  x : Outport
  wires:
  Q/1 -> "Complex Multiplier 3.1 "/2, Delay/1
  Delay/1 -> Negate/1
  Delay1/1 -> "Complex Multiplier 3.1 "/3
  Negate/1 -> "Complex Multiplier 3.1 "/4
  "Complex Multiplier 3.1 "/1 -> CORDIC ATAN/1(x)
  "Complex Multiplier 3.1 "/2 -> CORDIC ATAN/2(y)
  CORDIC ATAN/1(X) -> Terminator/1
  MSB/1 -> Inverter/1
  Inverter/1 -> Down Sample/1
  CORDIC ATAN/2(Z) -> MSB/1
  Down Sample/1 -> x/1
  I/1 -> "Complex Multiplier 3.1 "/1, Delay1/1

== system receiver_overall_reset/Receiver/PSDU length ==
  now : Inport
  data : Inport  Port=2
  AddSub : xbsIndex_r4/AddSub  mode=Addition  use_carryin=off  use_carryout=off  en=off  latency=0  precision=Full  arith_type=Unsigned  n_bits=16  bin_pt=14  quantization=Truncate  overflow=Wrap  dbl_ovrd=off  use_behavioral_HDL=off  hw_selection=Fabric  pipelined=off  block_type=addsub
      settings: block_version=12.2
  Constant : xbsIndex_r4/Constant  arith_type=Unsigned  const=0  n_bits=7  bin_pt=0  explicit_period=off  period=1  equ=P=C  opselect=C  inp2=PCIN>>17  opr=+  inp1=P  carry=CIN  dbl_ovrd=off  block_type=constant
      settings: block_version=12.2
  Constant1 : xbsIndex_r4/Constant  arith_type=Signed (2's comp)  const=1  n_bits=16  bin_pt=14  explicit_period=off  period=1  equ=P=C  opselect=C  inp2=PCIN>>17  opr=+  inp1=P  carry=CIN  dbl_ovrd=off  block_type=constant
      settings: block_version=12.2
  PSDU length : xbsIndex_r4/Mux  inputs=2  en=off  latency=0  precision=User Defined  arith_type=Unsigned  n_bits=8  bin_pt=0  quantization=Truncate  overflow=Wrap  dbl_ovrd=off  block_type=mux
      settings: block_version=12.2
  length : Outport
  wires:
  Constant/1 -> PSDU length/2
  AddSub/1 -> PSDU length/3
  Constant1/1 -> AddSub/2
  now/1 -> PSDU length/1
  data/1 -> AddSub/1
  PSDU length/1 -> length/1

== system receiver_overall_reset/Receiver/SFD_d ==
  not running : Inport
  data : Inport  Port=2
  Logical : xbsIndex_r4/Logical  logical_function=AND  inputs=2  en=off  latency=0  precision=Full  arith_type=Unsigned  n_bits=16  bin_pt=0  align_bp=on  dbl_ovrd=off  block_type=logical
      settings: block_version=12.2
  SFD : xbsIndex_r4/Constant  arith_type=Unsigned  const=167  n_bits=8  bin_pt=0  explicit_period=off  period=1  equ=P=C  opselect=C  inp2=PCIN>>17  opr=+  inp1=P  carry=CIN  dbl_ovrd=off  block_type=constant
      settings: block_version=12.2
  isSFD : xbsIndex_r4/Relational  mode=a=b  en=off  latency=0  dbl_ovrd=off  block_type=relational
      settings: block_version=12.2
  fnd : Outport
  wires:
  SFD/1 -> isSFD/2
  isSFD/1 -> Logical/2
  data/1 -> isSFD/1
  not running/1 -> Logical/1
  Logical/1 -> fnd/1

== system receiver_overall_reset/Receiver/Sym-Chooser ==
  In : Inport
  clk : Inport  Port=2
  0-8 : Subsystem  mask{a=0, b=8, chip_a=1618456172}
      mask prompts: a "Symbol a"; b "Symbol b"; chip_a "Chipping seq. for a"
  1-9 : Subsystem  mask{a=1, b=9, chip_a=1309113062}
      mask prompts: a "Symbol a"; b "Symbol b"; chip_a "Chipping seq. for a"
  2-10 : Subsystem  mask{a=2, b=10, chip_a=1826650030}
      mask prompts: a "Symbol a"; b "Symbol b"; chip_a "Chipping seq. for a"
  3-11 : Subsystem  mask{a=3, b=11, chip_a=1724778362}
      mask prompts: a "Symbol a"; b "Symbol b"; chip_a "Chipping seq. for a"
  4-12 : Subsystem  mask{a=4, b=12, chip_a=778887287}
      mask prompts: a "Symbol a"; b "Symbol b"; chip_a "Chipping seq. for a"
  5-13 : Subsystem  mask{a=5, b=13, chip_a=2061946375}
      mask prompts: a "Symbol a"; b "Symbol b"; chip_a "Chipping seq. for a"
  6-14 : Subsystem  mask{a=6, b=14, chip_a=2007919840}
      mask prompts: a "Symbol a"; b "Symbol b"; chip_a "Chipping seq. for a"
  7-15 : Subsystem  mask{a=7, b=15, chip_a=125494990}
      mask prompts: a "Symbol a"; b "Symbol b"; chip_a "Chipping seq. for a"
  Concat : xbsIndex_r4/Concat  num_inputs=8  dbl_ovrd=off  block_type=concat
      settings: block_version=12.2
  Constant : xbsIndex_r4/Constant  arith_type=Signed (2's comp)  const=1  n_bits=16  bin_pt=14  explicit_period=off  period=1  equ=P=C  opselect=C  inp2=PCIN>>17  opr=+  inp1=P  carry=CIN  dbl_ovrd=off  block_type=constant
      settings: block_version=12.2
  Down Sample1 : xbsIndex_r4/Down Sample  sample_ratio=32  sample_phase="Last Value of Frame  (most efficient)"  en=off  latency=1  dbl_ovrd=off  block_type=dsamp
      settings: block_version=12.2
  Down Sample2 : xbsIndex_r4/Down Sample  sample_ratio=32  sample_phase="Last Value of Frame  (most efficient)"  en=off  latency=1  dbl_ovrd=off  block_type=dsamp
      settings: block_version=12.2
  Logical : xbsIndex_r4/Logical  logical_function=OR  inputs=8  en=off  latency=0  precision=Full  arith_type=Unsigned  n_bits=4  bin_pt=0  align_bp=on  dbl_ovrd=off  block_type=logical
      settings: xl_area=[10 0 0 15 0 0 0]  block_version=12.1
  Logical1 : xbsIndex_r4/Logical  logical_function=OR  inputs=8  en=off  latency=0  precision=Full  arith_type=Unsigned  n_bits=4  bin_pt=0  align_bp=on  dbl_ovrd=off  block_type=logical
      settings: xl_area=[10 0 0 15 0 0 0]  block_version=12.1
  Relational{,1..7} (8 alike) : xbsIndex_r4/Relational  mode=a=b  en=off  latency=0  dbl_ovrd=off  block_type=relational
      settings: block_version=12.2
  Shift : xbsIndex_r4/Shift  shift_dir=Left  shift_bits=1  en=off  latency=0  precision=Full  arith_type="Signed  (2's comp)"  n_bits=16  bin_pt=14  quantization=Truncate  overflow=Wrap  dbl_ovrd=off  block_type=shift
      settings: block_version=12.2
  Shift1 : xbsIndex_r4/Shift  shift_dir=Left  shift_bits=2  en=off  latency=0  precision=Full  arith_type="Signed  (2's comp)"  n_bits=16  bin_pt=14  quantization=Truncate  overflow=Wrap  dbl_ovrd=off  block_type=shift
      settings: block_version=12.2
  Shift2 : xbsIndex_r4/Shift  shift_dir=Left  shift_bits=3  en=off  latency=0  precision=Full  arith_type="Signed  (2's comp)"  n_bits=16  bin_pt=14  quantization=Truncate  overflow=Wrap  dbl_ovrd=off  block_type=shift
      settings: block_version=12.2
  Shift3 : xbsIndex_r4/Shift  shift_dir=Left  shift_bits=4  en=off  latency=0  precision=Full  arith_type="Signed  (2's comp)"  n_bits=16  bin_pt=14  quantization=Truncate  overflow=Wrap  dbl_ovrd=off  block_type=shift
      settings: block_version=12.2
  Shift4 : xbsIndex_r4/Shift  shift_dir=Left  shift_bits=5  en=off  latency=0  precision=Full  arith_type="Signed  (2's comp)"  n_bits=16  bin_pt=14  quantization=Truncate  overflow=Wrap  dbl_ovrd=off  block_type=shift
      settings: block_version=12.2
  Shift5 : xbsIndex_r4/Shift  shift_dir=Left  shift_bits=6  en=off  latency=0  precision=Full  arith_type="Signed  (2's comp)"  n_bits=16  bin_pt=14  quantization=Truncate  overflow=Wrap  dbl_ovrd=off  block_type=shift
      settings: block_version=12.2
  Shift6 : xbsIndex_r4/Shift  shift_dir=Left  shift_bits=7  en=off  latency=0  precision=Full  arith_type="Signed  (2's comp)"  n_bits=16  bin_pt=14  quantization=Truncate  overflow=Wrap  dbl_ovrd=off  block_type=shift
      settings: block_version=12.2
  "[4:0]" : xbsIndex_r4/Slice  nbits=4  boolean_output=off  mode=Lower Bit Location + Width  bit1=0  base1=MSB of Input  bit0=0  base0=LSB of Input  dbl_ovrd=off  block_type=slice
      settings: block_version=12.1
  fnd : Outport
  symb : Outport  Port=2
  wires:
  clk/1 -> 1-9/2(clk), 0-8/2(clk), 2-10/2(clk), 3-11/2(clk), 4-12/2(clk), 5-13/2(clk), 6-14/2(clk), 7-15/2(clk)
  Down Sample2/1 -> symb/1
  7-15/2(value) -> Logical/8
  6-14/2(value) -> Logical/7
  5-13/2(value) -> Logical/6
  4-12/2(value) -> Logical/5
  3-11/2(value) -> Logical/4
  2-10/2(value) -> Logical/3
  1-9/2(value) -> Logical/2
  0-8/2(value) -> Logical/1
  0-8/1(fnd) -> Concat/1
  1-9/1(fnd) -> Concat/2
  2-10/1(fnd) -> Concat/3
  3-11/1(fnd) -> Concat/4
  4-12/1(fnd) -> Concat/5
  5-13/1(fnd) -> Concat/6
  6-14/1(fnd) -> Concat/7
  7-15/1(fnd) -> Concat/8
  In/1 -> 7-15/1(in), 6-14/1(in), 5-13/1(In), 4-12/1(in), 3-11/1(in), 2-10/1(In), 1-9/1(In), 0-8/1(in)
  Logical/1 -> "[4:0]"/1
  "[4:0]"/1 -> Down Sample2/1
  Down Sample1/1 -> fnd/1
  Concat/1 -> Relational/2, Relational1/2, Relational2/2, Relational3/2, Relational4/2, Relational5/2, Relational6/2, Relational7/2
  Shift5/1 -> Relational1/1
  Shift4/1 -> Relational2/1
  Shift3/1 -> Relational3/1
  Shift2/1 -> Relational4/1
  Shift1/1 -> Relational5/1
  Shift/1 -> Relational6/1
  Shift6/1 -> Relational/1
  Constant/1 -> Relational7/1, Shift/1, Shift1/1, Shift2/1, Shift3/1, Shift4/1, Shift5/1, Shift6/1
  Relational7/1 -> Logical1/8
  Relational6/1 -> Logical1/7
  Relational5/1 -> Logical1/6
  Relational4/1 -> Logical1/5
  Relational3/1 -> Logical1/4
  Relational2/1 -> Logical1/3
  Relational1/1 -> Logical1/2
  Relational/1 -> Logical1/1
  Logical1/1 -> Down Sample1/1
